simulink model "E2_SIM"  (R2025a)
settings: Solver=ode4  StartTime=0.0  StopTime=35  FixedStep=0.002  RelTol=1e-3  EnableMultiTasking=on
undefined symbols (not defined in the file): alpha_meas, mode, nis, ref, seq, theta_meas, Vm, xhat
libraries: simulink x1, quarc_library x1
settings Model: ExtModeTrigDuration=10000  Creator=sebas  LastModifiedBy=sebas
settings SolverCC: AlgebraicLoopSolver=TrustRegion  PositivePriorityOrder=on
settings DataIOCC: ReturnWorkspaceOutputs=off
settings DebuggingCC: UnconnectedInputMsg=warning  UnconnectedOutputMsg=warning  UnconnectedLineMsg=warning  ArithmeticOperatorsInVariantConditions=warning
settings HardwareCC: ProdHWDeviceType=AMD->x86-64 (Windows64)
settings ModelReferenceCC: EnableRefExpFcnMdlSchedulingChecks=on
settings SFSimCC: SimUseLocalCustomCode=off  CustomCodeUndefinedFunction=UseInterfaceOnly
settings RTWCC: SystemTargetFile=quarc_win64.tlc  TemplateMakefile=quarc_default_tmf  RTWUseLocalCustomCode=off  Toolchain=QUARC win64 | nmake (64-bit Windows)  BuildConfiguration=Faster Runs  GPUComputeCapability=3.5  Description=QUARC Win64 Target Using Toolchain
settings CodeAppCC: StateflowObjectComments=on
settings STFCustomTargetCC: SystemTargetFile=quarc_win64.tlc  TargetLangStandard=C99 (ISO)  MultiwordLength=2048.0  DynamicStringBufferSize=256.0  ConcurrentExecutionCompliant=on  UseToolchainInfoCompliant=on
settings GRTTargetCC: ExtMode=on  ExtModeMexFile=quarc_comm  ParMdlRefBuildCompliant=off  CompOptLevelCompliant=off  CombineOutputUpdateFcns=off  MatFileLogging=off  CPPClassGenCompliant=off  GRTInterface=on
settings ConfigComp: CovMetricSettings=dswe

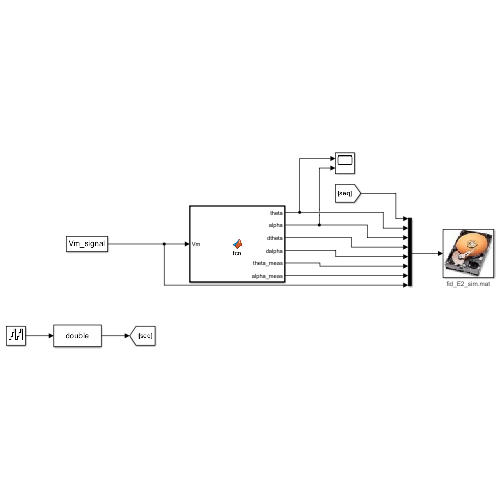
[thumbnail: Simulink's stored preview of the top-level diagram]
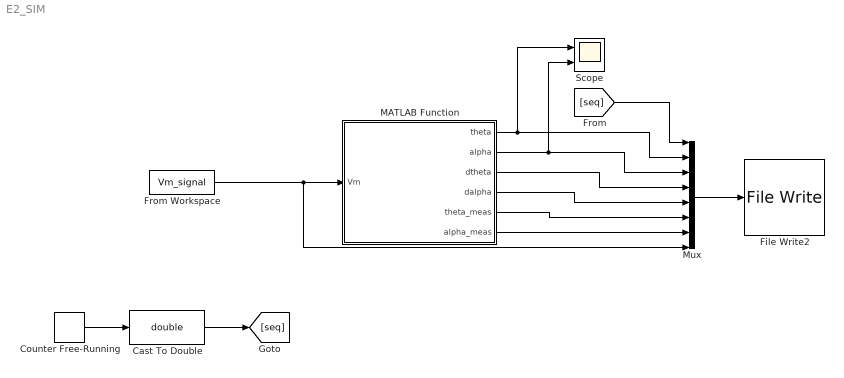
== system E2_SIM ==
  Cast To Double : DataTypeConversion  OutDataTypeStr=double  SaturateOnIntegerOverflow=off  RndMeth=Floor
  Counter Free-Running : simulink/Sources/Counter Free-Running  NumBits=16  tsamp=0.002
  File Write2 : quarc_library/Sinks/To Target/File Write  source=Specify via dialog (do not evaluate)  file_name=fid_E2_sim.mat  variable_name=seq,theta_meas,alpha_meas,Vm,xhat.dhat,nis,mode,E,ref  decimation=1  sample_time=0.002  file_format=MAT-file v.4  options=No header or footer  append=off  encoding=Default  bitrate=0
      settings: AttributesFormatString=%<file_name>  SourceProductName=QUARC Targets
  From Workspace : FromWorkspace  VariableName=Vm_signal  SampleTime=0.002  Interpolate=off  OutputAfterFinalValue=Holding final value
  MATLAB Function : MATLAB Function  TreatAsAtomicUnit=on
  Mux : Mux  Inputs=8
  Scope : Scope  NumInputPorts=2
      settings: ActiveDisplayYMinimum=-3.3554213197724083  ActiveDisplayYMaximum=6.4927493659376205
  wires:
  From Workspace/1 -> Mux/8, MATLAB Function/1(Vm)
  Mux/1 -> File Write2/1
  Cast To Double/1 -> [seq]
  Counter Free-Running/1 -> Cast To Double/1
  [seq] -> Mux/1
  MATLAB Function/1(theta) -> Scope/1, Mux/2
  MATLAB Function/2(alpha) -> Scope/2, Mux/3
  MATLAB Function/3(dtheta) -> Mux/4
  MATLAB Function/4(dalpha) -> Mux/5
  MATLAB Function/5(theta_meas) -> Mux/6
  MATLAB Function/6(alpha_meas) -> Mux/7

== matlab function E2_SIM/MATLAB Function ==
  data: Vm input; theta output; alpha output; dtheta output; dalpha output; theta_meas output; alpha_meas output
function [theta,alpha,dtheta,dalpha,theta_meas,alpha_meas] = fcn(Vm)
%#codegen
% E1: x0=[0;0.05;0;0]  |  E2 y E3: x0=[0;pi;0;0]
[theta,alpha,dtheta,dalpha,theta_meas,alpha_meas] = ...
    furuta_planta_analitica(Vm, [0;pi;0;0], 0.002, 4);
end
